simulink model "elec_bipolar_npn_optimised"  (R2018b)
settings: Solver=VariableStepAuto  StartTime=0.0  StopTime=0.04  RelTol=1e-3  AbsTol=1e-3  EnableMultiTasking=on
values from neighbouring files (symbols this model uses):
  fsw = n * 2e3    [Hysteresis.m]    (also in OPtimized.m; SVM.m)
  r = 3    [Hysteresis.m]    (also in OPtimized.m; SVM.m)
libraries: fl_lib x40, nesl_utility x29, elec_lib x12, powerlib_meascontrol x10, simulink x2
settings Model: Creator=Dr. Eskandari  LastModifiedBy=Iftikhw1
settings SolverCC: AutoScaleAbsTol=off
settings DataIOCC: LimitDataPoints=on
settings OptimizationCC: LifeSpan=inf
settings DebuggingCC: AllowSymbolicDim=off  SFUnexpectedBacktrackingDiag=warning  SFNoUnconditionalDefaultTransitionDiag=warning  SFExecutionAtInitializationDiag=none
settings SFSimCC: SimUseLocalCustomCode=off
settings RTWCC: RTWUseLocalCustomCode=off
settings CodeAppCC: StateflowObjectComments=on
settings GRTTargetCC: TargetLangStandard=C89/C90 (ANSI)  GeneratePreprocessorConditionals=Disable all
settings ConfigComp: CovMetricSettings=dw  CovHtmlReporting=on  CovSaveCumulativeToWorkspaceVar=on  CovSaveSingleToWorkspaceVar=on  CovExternalEMLEnable=off  CovSFcnEnable=off
settings SimscapeCC: SimscapeNormalizeSystem=off  SimscapeLogType=all  SimscapeLogDataHistory=10000

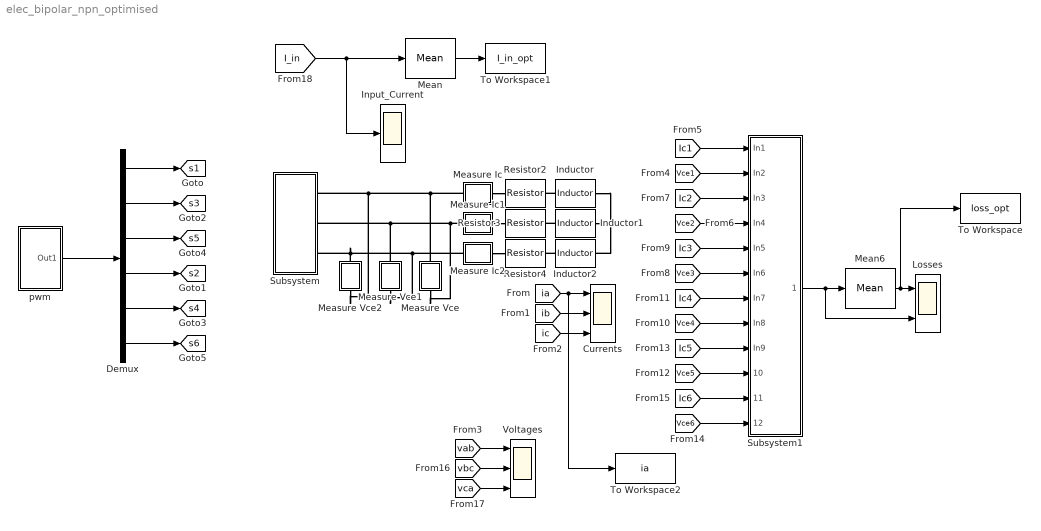
== system elec_bipolar_npn_optimised ==
  Currents : Scope  NumInputPorts=3
  Demux : Demux  Outputs=6
  Inductor : fl_lib/Electrical/Electrical Elements/Inductor  l=1000e-6 H  r=0 Ohm  g=1e-9 1/Ohm  i_specify=off  i_priority=None  i=0 A  i_nominal_specify=off  i_nominal_unit=A  i_nominal_value=1  v_specify=off  v_priority=None  v=0 V  v_nominal_specify=off  v_nominal_unit=V  v_nominal_value=1  i_L_specify=off  i_L_priority=High  i_L=0 A  i_L_nominal_specify=off  i_L_nominal_unit=A  i_L_nominal_value=1
  Inductor1 : fl_lib/Electrical/Electrical Elements/Inductor  l=1000e-6 H  r=0 Ohm  g=1e-9 1/Ohm  i_specify=off  i_priority=None  i=0 A  i_nominal_specify=off  i_nominal_unit=A  i_nominal_value=1  v_specify=off  v_priority=None  v=0 V  v_nominal_specify=off  v_nominal_unit=V  v_nominal_value=1  i_L_specify=off  i_L_priority=High  i_L=0 A  i_L_nominal_specify=off  i_L_nominal_unit=A  i_L_nominal_value=1
  Inductor2 : fl_lib/Electrical/Electrical Elements/Inductor  l=1000e-6 H  r=0 Ohm  g=1e-9 1/Ohm  i_specify=off  i_priority=None  i=0 A  i_nominal_specify=off  i_nominal_unit=A  i_nominal_value=1  v_specify=off  v_priority=None  v=0 V  v_nominal_specify=off  v_nominal_unit=V  v_nominal_value=1  i_L_specify=off  i_L_priority=High  i_L=0 A  i_L_nominal_specify=off  i_L_nominal_unit=A  i_L_nominal_value=1
  Input_Current : Scope
  Losses : Scope  NumInputPorts=2
  Mean : powerlib_meascontrol/Measurements/Mean  Freq=fsw  Vinit=0  Ts=0
  Mean6 : powerlib_meascontrol/Measurements/Mean  Freq=150  Vinit=0  Ts=0
      settings: SourceProductName=Simscape Electrical
  Measure Ic : Subsystem
  Measure Ic1 : Subsystem
  Measure Ic2 : Subsystem
  Measure Vce : Subsystem
  Measure Vce1 : Subsystem
  Measure Vce2 : Subsystem
  Resistor2 : fl_lib/Electrical/Electrical Elements/Resistor  R=r Ohm  i_specify=off  i_priority=None  i=0 A  i_nominal_specify=off  i_nominal_unit=A  i_nominal_value=1  v_specify=off  v_priority=None  v=0 V  v_nominal_specify=off  v_nominal_unit=V  v_nominal_value=1
  Resistor3 : fl_lib/Electrical/Electrical Elements/Resistor  R=r Ohm  i_specify=off  i_priority=None  i=0 A  i_nominal_specify=off  i_nominal_unit=A  i_nominal_value=1  v_specify=off  v_priority=None  v=0 V  v_nominal_specify=off  v_nominal_unit=V  v_nominal_value=1
  Resistor4 : fl_lib/Electrical/Electrical Elements/Resistor  R=r Ohm  i_specify=off  i_priority=None  i=0 A  i_nominal_specify=off  i_nominal_unit=A  i_nominal_value=1  v_specify=off  v_priority=None  v=0 V  v_nominal_specify=off  v_nominal_unit=V  v_nominal_value=1
  Subsystem : Subsystem
  Subsystem1 : Subsystem
  To Workspace : ToWorkspace  VariableName=loss_opt  SampleTime=-1
      settings: MaxDataPoints=1
  To Workspace1 : ToWorkspace  VariableName=I_in_opt  SampleTime=-1
      settings: MaxDataPoints=1
  To Workspace2 : ToWorkspace  VariableName=ia  SampleTime=-1
      settings: MaxDataPoints=1
  Voltages : Scope  NumInputPorts=3
  pwm : Subsystem
  tag scope: s1=global, s2=global, s3=global, s4=global, s5=global, s6=global
  wires:
  Demux/1 -> [s1]
  [ia] -> To Workspace2/1, Currents/1
  [ib] -> Currents/2
  [ic] -> Currents/3
  Mean6/1 -> To Workspace/1, Losses/1
  [Ic1] -> Subsystem1/1(In1)
  [Vce1] -> Subsystem1/2(In2)
  [Ic2] -> Subsystem1/3(In3)
  [Vce2] -> Subsystem1/4(In4)
  [Ic3] -> Subsystem1/5(In5)
  [Vce3] -> Subsystem1/6(In6)
  [Ic4] -> Subsystem1/7(In7)
  [Vce4] -> Subsystem1/8(In8)
  [Ic5] -> Subsystem1/9(In9)
  [Vce5] -> Subsystem1/10(In10)
  [Ic6] -> Subsystem1/11(In11)
  [Vce6] -> Subsystem1/12(In12)
  Subsystem1/1(Out1) -> Losses/2, Mean6/1
  pwm/1(Out1) -> Demux/1
  Demux/4 -> [s2]
  Demux/2 -> [s3]
  Demux/5 -> [s4]
  Demux/3 -> [s5]
  Demux/6 -> [s6]
  [vca] -> Voltages/3
  [vbc] -> Voltages/2
  [vab] -> Voltages/1
  [I_in] -> Input_Current/1, Mean/1
  Mean/1 -> To Workspace1/1
  connections:
  Measure Ic/RConn1 -- Measure Vce/LConn1 -- Measure Vce2/RConn1 -- Subsystem/RConn1
  Measure Ic/LConn1 -- Resistor2/LConn1
  Measure Ic1/RConn1 -- Measure Vce/RConn1 -- Measure Vce1/LConn1 -- Subsystem/RConn2
  Measure Ic1/LConn1 -- Resistor3/LConn1
  Measure Ic2/RConn1 -- Measure Vce1/RConn1 -- Measure Vce2/LConn1 -- Subsystem/RConn3
  Measure Ic2/LConn1 -- Resistor4/LConn1
  Inductor/LConn1 -- Resistor2/RConn1
  Inductor1/LConn1 -- Resistor3/RConn1
  Inductor2/LConn1 -- Resistor4/RConn1
  Inductor/RConn1 -- Inductor1/RConn1 -- Inductor2/RConn1

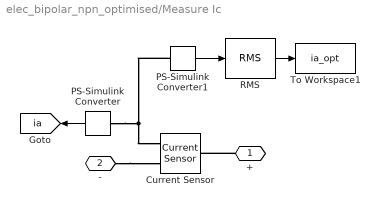
== system elec_bipolar_npn_optimised/Measure Ic ==
  Current Sensor : fl_lib/Electrical/Electrical Sensors/Current Sensor
  PS-Simulink Converter : nesl_utility/PS-Simulink Converter  PhysicalDomain=network_engine_domain  SubClassName=ps_output  LeftPortType=input  RightPortType=output  PseudoPeriodic=off  Frequencies=[]  Unit=1  AffineConversion=off
  PS-Simulink Converter1 : nesl_utility/PS-Simulink Converter  PhysicalDomain=network_engine_domain  SubClassName=ps_output  LeftPortType=input  RightPortType=output  PseudoPeriodic=off  Frequencies=[]  Unit=1  AffineConversion=off
  RMS : powerlib_meascontrol/Measurements/RMS  TrueRMS=off  Freq=50  RMSInit=0  Ts=0
  To Workspace1 : ToWorkspace  VariableName=ia_opt  SampleTime=-1
  + : PMIOPort  Side=Left
  - : PMIOPort  Port=2  Side=Right
  tag scope: ia=global
  wires:
  PS-Simulink Converter/1 -> [ia]
  PS-Simulink Converter1/1 -> RMS/1
  RMS/1 -> To Workspace1/1
  connections:
  +/RConn1 -- Current Sensor/LConn1
  -/RConn1 -- Current Sensor/RConn2
  PS-Simulink Converter/LConn1 -- Current Sensor/RConn1 -- PS-Simulink Converter1/LConn1

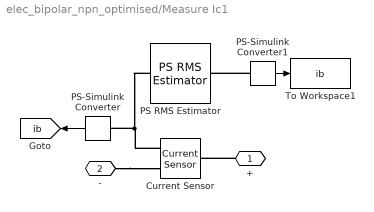
== system elec_bipolar_npn_optimised/Measure Ic1 ==
  Current Sensor : fl_lib/Electrical/Electrical Sensors/Current Sensor
  PS RMS Estimator : fl_lib/Physical Signals/Periodic Operators/PS RMS Estimator  f0=50 Hz
      settings: SourceProductName=Simscape  SourceProductBaseCode=SS
  PS-Simulink Converter : nesl_utility/PS-Simulink Converter  PhysicalDomain=network_engine_domain  SubClassName=ps_output  LeftPortType=input  RightPortType=output  PseudoPeriodic=off  Frequencies=[]  Unit=1  AffineConversion=off
  PS-Simulink Converter1 : nesl_utility/PS-Simulink Converter  PhysicalDomain=network_engine_domain  SubClassName=ps_output  LeftPortType=input  RightPortType=output  PseudoPeriodic=off  Frequencies=[]  Unit=1  AffineConversion=off
  To Workspace1 : ToWorkspace  VariableName=ib  SaveFormat=Timeseries  SampleTime=-1
  + : PMIOPort  Side=Left
  - : PMIOPort  Port=2  Side=Right
  tag scope: ib=global
  wires:
  PS-Simulink Converter/1 -> [ib]
  PS-Simulink Converter1/1 -> To Workspace1/1
  connections:
  Current Sensor/RConn1 -- PS RMS Estimator/LConn1 -- PS-Simulink Converter/LConn1
  -/RConn1 -- Current Sensor/RConn2
  +/RConn1 -- Current Sensor/LConn1
  PS-Simulink Converter1/LConn1 -- PS RMS Estimator/RConn1

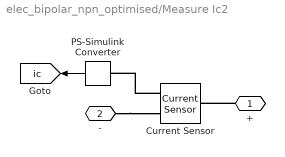
== system elec_bipolar_npn_optimised/Measure Ic2 ==
  Current Sensor : fl_lib/Electrical/Electrical Sensors/Current Sensor
  PS-Simulink Converter : nesl_utility/PS-Simulink Converter  PhysicalDomain=network_engine_domain  SubClassName=ps_output  LeftPortType=input  RightPortType=output  PseudoPeriodic=off  Frequencies=[]  Unit=1  AffineConversion=off
  + : PMIOPort  Side=Left
  - : PMIOPort  Port=2  Side=Right
  tag scope: ic=global
  wires:
  PS-Simulink Converter/1 -> [ic]
  connections:
  +/RConn1 -- Current Sensor/LConn1
  -/RConn1 -- Current Sensor/RConn2
  Current Sensor/RConn1 -- PS-Simulink Converter/LConn1

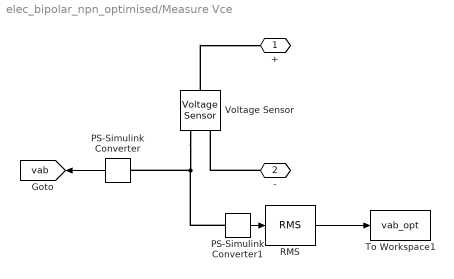
== system elec_bipolar_npn_optimised/Measure Vce ==
  PS-Simulink Converter : nesl_utility/PS-Simulink Converter  PhysicalDomain=network_engine_domain  SubClassName=ps_output  LeftPortType=input  RightPortType=output  PseudoPeriodic=off  Frequencies=[]  Unit=V  AffineConversion=off
  PS-Simulink Converter1 : nesl_utility/PS-Simulink Converter  PhysicalDomain=network_engine_domain  SubClassName=ps_output  LeftPortType=input  RightPortType=output  PseudoPeriodic=off  Frequencies=[]  Unit=1  AffineConversion=off
  RMS : powerlib_meascontrol/Measurements/RMS  TrueRMS=off  Freq=50  RMSInit=0  Ts=0
  To Workspace1 : ToWorkspace  VariableName=vab_opt  SampleTime=-1
  Voltage Sensor : fl_lib/Electrical/Electrical Sensors/Voltage Sensor
  + : PMIOPort  Side=Left
  - : PMIOPort  Port=2  Side=Right
  tag scope: vab=global
  wires:
  PS-Simulink Converter/1 -> [vab]
  PS-Simulink Converter1/1 -> RMS/1
  RMS/1 -> To Workspace1/1
  connections:
  Voltage Sensor/LConn1 -- +/RConn1
  -/RConn1 -- Voltage Sensor/RConn2
  Voltage Sensor/RConn1 -- PS-Simulink Converter1/LConn1 -- PS-Simulink Converter/LConn1

== system elec_bipolar_npn_optimised/Measure Vce1 ==
  PS-Simulink Converter : nesl_utility/PS-Simulink Converter  PhysicalDomain=network_engine_domain  SubClassName=ps_output  LeftPortType=input  RightPortType=output  PseudoPeriodic=off  Frequencies=[]  Unit=V  AffineConversion=off
  Voltage Sensor : fl_lib/Electrical/Electrical Sensors/Voltage Sensor
  + : PMIOPort  Side=Left
  - : PMIOPort  Port=2  Side=Right
  tag scope: vbc=global
  wires:
  PS-Simulink Converter/1 -> [vbc]
  connections:
  Voltage Sensor/RConn1 -- PS-Simulink Converter/LConn1
  -/RConn1 -- Voltage Sensor/RConn2
  Voltage Sensor/LConn1 -- +/RConn1

== system elec_bipolar_npn_optimised/Measure Vce2 ==
  PS-Simulink Converter : nesl_utility/PS-Simulink Converter  PhysicalDomain=network_engine_domain  SubClassName=ps_output  LeftPortType=input  RightPortType=output  PseudoPeriodic=off  Frequencies=[]  Unit=V  AffineConversion=off
  Voltage Sensor : fl_lib/Electrical/Electrical Sensors/Voltage Sensor
  + : PMIOPort  Side=Left
  - : PMIOPort  Port=2  Side=Right
  tag scope: vca=global
  wires:
  PS-Simulink Converter/1 -> [vca]
  connections:
  Voltage Sensor/LConn1 -- +/RConn1
  -/RConn1 -- Voltage Sensor/RConn2
  Voltage Sensor/RConn1 -- PS-Simulink Converter/LConn1

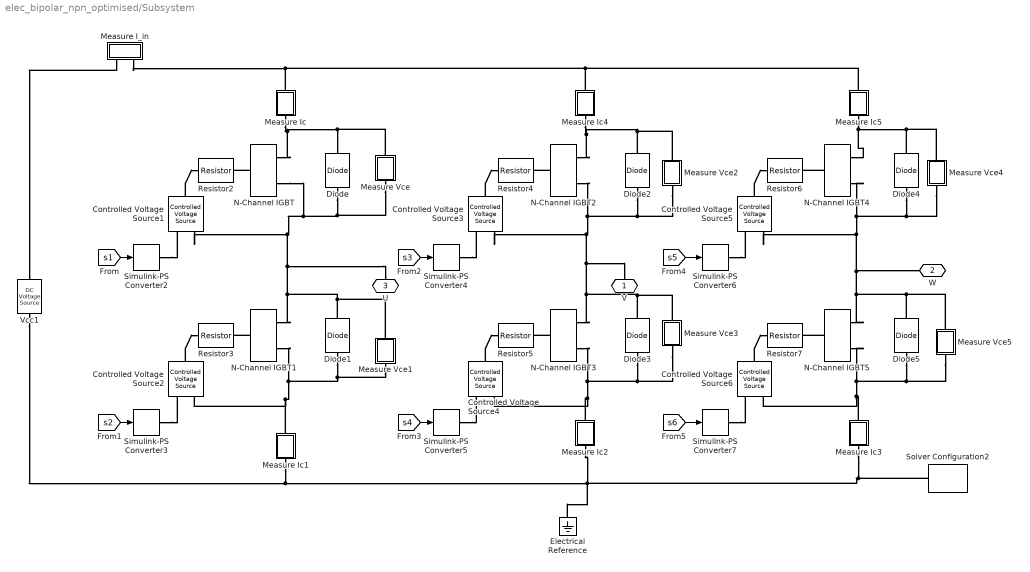
== system elec_bipolar_npn_optimised/Subsystem ==
  Controlled Voltage Source{1..6} (6 alike) : fl_lib/Electrical/Electrical Sources/Controlled Voltage Source
  Diode{,1..5} (6 alike) : elec_lib/Semiconductor Devices/Diode  ModelType=1  Vf=2.15 V  Ron=0.0063 Ohm  Goff=1e-8 S  Rz=0.3 Ohm  Vz=50 V  C_PWL=5 pF  prmExp=1  I12=[ 0.0137 0.545 ] A  V12=[ 0.6 0.7 ] V  I1=0.0137 A  V1=0.6 V  IS=1e-12 A  ec=1  RS=0.01 Ohm  Tmeas=25 degC  BV=Inf V  C_param=1  CJ0=5 pF  VJ=1 V  Mgrad=0.5  Vvec=[ 0.1 10 100 ] V  Cvec=[ 3.5 1 0.4 ] pF  FC=0.5  Q_param=1  Irrm=-7.15 A  iF=4 A  didt=-750 A/us  trr=115 ns  TT=50 ns  tau=100 ns  T_param=1  IS_T2=1.25e-7 A  I1_T2=0.245 A  V1_T2=0.5 V  Tmeas2=125 degC  EG_param=1  EG=1.11 eV  XTI_param=1  XTI=3  dBVdT=0 V/K  Tdevice=25 degC  i_capacitor_specify=off  i_capacitor_priority=High  i_capacitor=0 A  i_capacitor_nominal_specify=off  i_capacitor_nominal_unit=A  i_capacitor_nominal_value=1  v_capacitor_specify=off  v_capacitor_priority=None  v_capacitor=0 V  v_capacitor_nominal_specify=off  v_capacitor_nominal_unit=V  v_capacitor_nominal_value=1  Rth=[ 0 10 ] K/W  thermal_mass_parameterization=1  thermal_mass=[ 0 1 ] J/K  thermal_time_constant=[ 0 10 ] s  thermal_mass_initial_temperatures=[ 25 25 ] degC
      settings: SourceProductName=Simscape Electronics  SourceProductBaseCode=SN
  Electrical Reference : fl_lib/Electrical/Electrical Elements/Electrical Reference
  Measure Ic : Subsystem
  Measure Ic1 : Subsystem
  Measure Ic2 : Subsystem
  Measure Ic3 : Subsystem
  Measure Ic4 : Subsystem
  Measure Ic5 : Subsystem
  Measure Vce : Subsystem
  Measure Vce1 : Subsystem
  Measure Vce2 : Subsystem
  Measure Vce3 : Subsystem
  Measure Vce4 : Subsystem
  Measure Vce5 : Subsystem
  Measure I_in : Subsystem
  N-Channel IGBT{,1..5} (6 alike) : elec_lib/Semiconductor Devices/N-Channel IGBT  model_type=1  Ices=2.6 mA  Vces=1200 V  Vth=5.8 V  Vce_sat=2.05 V  Ice_sat=200 A  Vge_sat=15 V  ec=1  Tmeas=150 degC  Vge_vec=[ -2 6 7 8 10 12 15 20 ] V  Vce_vec=[ -1 0 0.5 1 1.5 2 2.5 3 3.5 4 ] V  T_vec=[25, 125] degC  Ic_mat=[ -1.015e-5 1.35e-8 4.7135e-4 5.092e-4 5.105e-4 5.117500000000001e-4 5.1299e-4 5.1423e-4 5.1548e-4 5.1672e-4; -9.986899999999999e-6 1.35e-8 4.7135e-4 5.092e-4 5.105e-4 5.117500000000001e-4 5.1299e-4 5.1423e-4 5.1548e-4 5.1672e-4; -9.955e-6 1.35e-8 0.0065225 3.3324 48.154 93.661 105.52 105.72 105.93 106.14; -9.955e-6 1.35e-8 0.0065235 3.5783 70.264 166.33 252.4 317.67 353.38 357.39; -9.955e-6 1.35e-8 0.006524 3.7206 89.17100000000001 228.09 371.63 511.02 642.6900000000001 764.04; -9.9549e-6 1.35e-8 0.0065242 3.7716 97.79300000000001 256.21 424.27 592.92 759.2 921.52; -9.9549e-6 1.35e-8 0.0065243 3.8067 104.52 278.11 464.6 654.37 844.5700000000001 1.0339e+3; -9.9549e-6 1.35e-8 0.0065244 3.8324 109.92 295.67 496.54 702.28 909.96 1.1183e+3 ] A  Ic_mat_3D=zeros(8, 10, 2) A  C_param=1  C_GE=23.7 nF  C_GC=2.7 nF  C_CE=0 nF  C_ies=12.5 nF  C_res=0.68 nF  C_oes=0.78 nF  C_GE_vec=[ 25 31 26.5 24.9 25 24.9 24.6 24.7 24.8 ] nF  C_GC_vec=[ 55 9 5.5 3.1 2.5 2.1 1.9 1.8 1.7 ] nF  C_CE_vec=[ 5 11 6.5 4.9 3.5 2.7 2.1 1.7 1.4 ] nF  C_ies_vec=[ 80 40 32 28 27.5 27 26.5 26.5 26.5 ] nF  C_res_vec=[ 55 9 5.5 3.1 2.5 2.1 1.9 1.8 1.7 ] nF  C_oes_vec=[ 60 20 12 8 6 4.8 4 3.5 3.1 ] nF  C_Vce_vec=[ 0 1 2 5 10 15 20 25 30 ] V  charge_linearity_param=1  C_OX=20 nF  V_C_OX=-5 V  TF=82 ns  VAF=200 V  RC=0.001 Ohm  RE=0.001 Ohm  RG=0.001 Ohm  BF=50  T_param=1  Ices_T2=100 mA  EG=1.11 eV  Vce_sat_T2=2.05 V  Tmeas2=150 degC  XTI=3  BEX=-1.5  RG_alpha=0 1/K  Tdevice=25 degC  Tdevice_3D=25 degC  Rth=[0.0, 10.0] K/W  thermal_mass_parameterization=1  thermal_mass=[0.0, 1.0] J/K  thermal_time_constant=[0.0, 10.0] s  thermal_mass_initial_temperatures=[298.15, 298.15] K  Ic_vec1=[0.0, 10.0, 50.0, 100.0, 200.0, 400.0, 600.0] A  Vce_vec1=[0.0, 1.1, 1.3, 1.45, 1.75, 2.25, 2.7] V  Rmiller=0.1 Ohm  Goff=1e-5 1/Ohm  t_on=0.07 us  t_rise=0.7 us  t_off=0.2 us  t_fall=0.5 us  v_meas=300 V  Tj_vec1=[298.15, 398.15] K  Vce_mat1=[0.0, 1.1, 1.3, 1.45, 1.75, 2.25, 2.7; 0.0, 1.0, 1.15, 1.35, 1.7, 2.35, 3.0] V  E_turn_on_mat1=[0.0, 0.2, 1.0, 2.0, 4.0, 8.0, 15.0; 0.0, 0.3, 1.3, 2.5, 5.0, 11.0, 18.0] * 1e-3 J  E_turn_off_mat1=[0.0, 0.3, 1.5, 3.0, 6.0, 15.0, 25.0; 0.0, 0.7, 3.3, 6.5, 13.0, 25.0, 35.0] * 1e-3 J
      settings: SourceProductName=Simscape Electronics  SourceProductBaseCode=SN
  Resistor{2..7} (6 alike) : fl_lib/Electrical/Electrical Elements/Resistor  R=3 Ohm  i_specify=off  i_priority=None  i=0 A  i_nominal_specify=off  i_nominal_unit=A  i_nominal_value=1  v_specify=off  v_priority=None  v=0 V  v_nominal_specify=off  v_nominal_unit=V  v_nominal_value=1
  Simulink-PS Converter{2..7} (6 alike) : nesl_utility/Simulink-PS Converter  PhysicalDomain=network_engine_domain  SubClassName=ps_input  LeftPortType=input  RightPortType=output  PseudoPeriodic=off  Frequencies=[]  NoiseDistribution=none  NoiseParameters=[]  Unit=V  AffineConversion=on  FilteringAndDerivatives=zero  SimscapeFilterOrder=1  InputFilterTimeConstant=.001  UdotUserProvided=1
  Solver Configuration2 : nesl_utility/Solver Configuration  PhysicalDomain=network_engine_domain  SubClassName=solver  LeftPortType=input  RightPortType=generic  Tones=[]  Harmonics=[]  SimulateNoise=off  Profile=off  UseLocalSampling=off  EnableSwitchedLinearOptims=on  FrequencyDomain=off  UseCCode=off  RelTol=0.001  AbsTol=1e-06  MinStep=1e-09  ToWorkspace=off  RevertToSquareIcSolve=off  NumHomotopyIterations=100  PhasorMode=off  PhasorModeNumHarmonics=1  DoDC=on  ResidualTolerance=1e-9  UseLocalSolver=on  LocalSolverChoice=NE_TRAPEZOIDAL_ADVANCER  LocalSolverSampleTime=0.00000001  DoFixedCost=off  MaxNonlinIter=3  MaxModeIter=2  LinearAlgebra=Sparse  EquationFormulation=NE_TIME_EF  DelaysMemoryBudget=1024  AutomaticFiltering=on  FilteringTimeConstant=0.001  PartitionStorageMethod=AS_NEEDED  PartitionMemoryBudget=1024
  Vcc1 : fl_lib/Electrical/Electrical Sources/DC Voltage Source  v0=540 V
  V : PMIOPort  Side=Right
  W : PMIOPort  Port=2  Side=Right
  U : PMIOPort  Port=3  Side=Right
  wires:
  [s1] -> Simulink-PS Converter2/1
  [s6] -> Simulink-PS Converter7/1
  [s2] -> Simulink-PS Converter3/1
  [s3] -> Simulink-PS Converter4/1
  [s4] -> Simulink-PS Converter5/1
  [s5] -> Simulink-PS Converter6/1
  connections:
  Simulink-PS Converter2/RConn1 -- Controlled Voltage Source1/RConn1
  N-Channel IGBT/LConn1 -- Resistor2/RConn1
  Measure Vce2/RConn1 -- Diode2/LConn1 -- N-Channel IGBT2/RConn2 -- V/RConn1 -- N-Channel IGBT3/RConn1 -- Diode3/RConn1 -- Measure Vce3/LConn1 -- Controlled Voltage Source3/RConn2
  Simulink-PS Converter5/RConn1 -- Controlled Voltage Source4/RConn1
  N-Channel IGBT3/LConn1 -- Resistor5/RConn1
  Controlled Voltage Source4/LConn1 -- Resistor5/LConn1
  Simulink-PS Converter4/RConn1 -- Controlled Voltage Source3/RConn1
  Controlled Voltage Source3/LConn1 -- Resistor4/LConn1
  N-Channel IGBT2/LConn1 -- Resistor4/RConn1
  Controlled Voltage Source1/LConn1 -- Resistor2/LConn1
  Controlled Voltage Source2/LConn1 -- Resistor3/LConn1
  N-Channel IGBT1/LConn1 -- Resistor3/RConn1
  Simulink-PS Converter3/RConn1 -- Controlled Voltage Source2/RConn1
  N-Channel IGBT4/LConn1 -- Resistor6/RConn1
  Controlled Voltage Source5/LConn1 -- Resistor6/LConn1
  N-Channel IGBT3/RConn2 -- Diode3/LConn1 -- Measure Vce3/RConn1 -- Measure Ic2/LConn1 -- Controlled Voltage Source4/RConn2
  Simulink-PS Converter6/RConn1 -- Controlled Voltage Source5/RConn1
  Controlled Voltage Source6/LConn1 -- Resistor7/LConn1
  N-Channel IGBT5/LConn1 -- Resistor7/RConn1
  Simulink-PS Converter7/RConn1 -- Controlled Voltage Source6/RConn1
  Measure Ic/LConn1 -- Measure I_in/RConn2 -- Measure Ic5/LConn1 -- Measure Ic4/LConn1
  Diode4/LConn1 -- Measure Vce4/RConn1 -- N-Channel IGBT4/RConn2 -- W/RConn1 -- N-Channel IGBT5/RConn1 -- Diode5/RConn1 -- Measure Vce5/LConn1 -- Controlled Voltage Source5/RConn2
  Measure Vce1/LConn1 -- Diode1/RConn1 -- N-Channel IGBT1/RConn1 -- U/RConn1 -- N-Channel IGBT/RConn2 -- Measure Vce/RConn1 -- Diode/LConn1 -- Controlled Voltage Source1/RConn2
  Measure Ic/RConn1 -- N-Channel IGBT/RConn1 -- Measure Vce/LConn1 -- Diode/RConn1
  Diode1/LConn1 -- Measure Vce1/RConn1 -- N-Channel IGBT1/RConn2 -- Measure Ic1/LConn1 -- Controlled Voltage Source2/RConn2
  Vcc1/RConn1 -- Measure Ic1/RConn1 -- Measure Ic3/RConn1 -- Solver Configuration2/RConn1 -- Measure Ic2/RConn1 -- Electrical Reference/LConn1
  Diode5/LConn1 -- Measure Vce5/RConn1 -- N-Channel IGBT5/RConn2 -- Measure Ic3/LConn1 -- Controlled Voltage Source6/RConn2
  Measure Ic4/RConn1 -- N-Channel IGBT2/RConn1 -- Diode2/RConn1 -- Measure Vce2/LConn1
  Measure Ic5/RConn1 -- N-Channel IGBT4/RConn1 -- Diode4/RConn1 -- Measure Vce4/LConn1
  Measure I_in/RConn1 -- Vcc1/LConn1

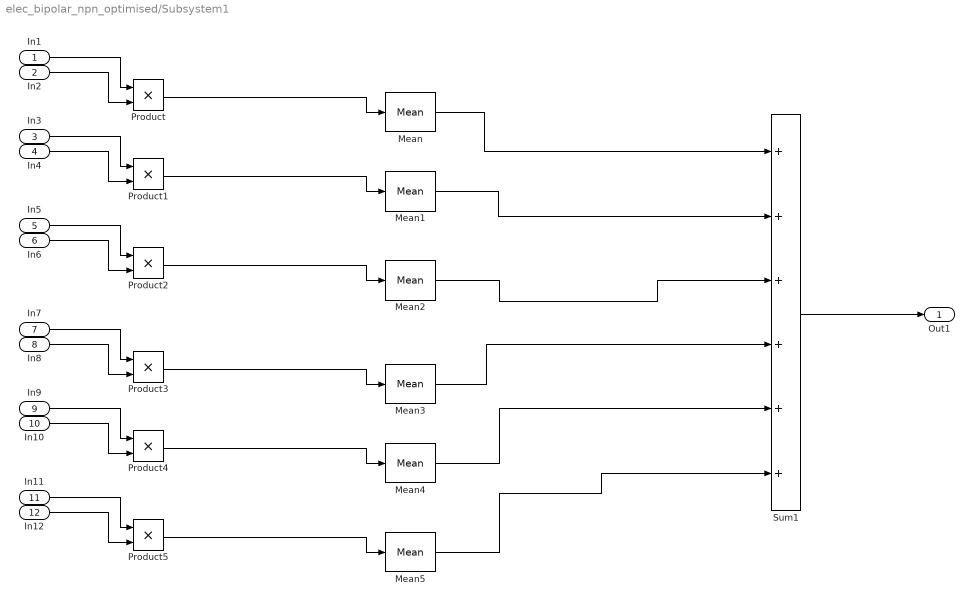
== system elec_bipolar_npn_optimised/Subsystem1 ==
  In1 : Inport
  In2 : Inport  Port=2
  In3 : Inport  Port=3
  In4 : Inport  Port=4
  In5 : Inport  Port=5
  In6 : Inport  Port=6
  In7 : Inport  Port=7
  In8 : Inport  Port=8
  In9 : Inport  Port=9
  In10 : Inport  Port=10
  In11 : Inport  Port=11
  In12 : Inport  Port=12
  Mean{,1..5} (6 alike) : powerlib_meascontrol/Measurements/Mean  Freq=fsw/2  Vinit=0  Ts=0
      settings: SourceProductName=Simscape Electrical
  Product{,1..5} (6 alike) : Product
  Sum1 : Sum  Inputs=++++++
  Out1 : Outport
  wires:
  Product/1 -> Mean/1
  In2/1 -> Product/2
  In1/1 -> Product/1
  Mean/1 -> Sum1/1
  Mean5/1 -> Sum1/6
  Mean1/1 -> Sum1/2
  Product5/1 -> Mean5/1
  In10/1 -> Product4/2
  In4/1 -> Product1/2
  Mean3/1 -> Sum1/4
  In9/1 -> Product4/1
  Mean2/1 -> Sum1/3
  In6/1 -> Product2/2
  In12/1 -> Product5/2
  Product1/1 -> Mean1/1
  In8/1 -> Product3/2
  Product2/1 -> Mean2/1
  Product3/1 -> Mean3/1
  In3/1 -> Product1/1
  In5/1 -> Product2/1
  Mean4/1 -> Sum1/5
  In11/1 -> Product5/1
  In7/1 -> Product3/1
  Sum1/1 -> Out1/1
  Product4/1 -> Mean4/1

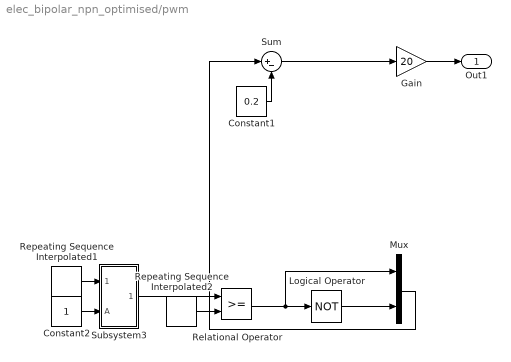
== system elec_bipolar_npn_optimised/pwm ==
  Constant1 : Constant  Value=0.2
  Constant2 : Constant
  Gain : Gain  Gain=20
  Logical Operator : Logic  Operator=NOT  AllPortsSameDT=off  OutDataTypeStr=boolean
  Mux : Mux  Inputs=2
  Relational Operator : RelationalOperator  OutDataTypeStr=boolean  RndMeth=Simplest
  Repeating Sequence Interpolated1 : simulink/Sources/Repeating Sequence Interpolated  OutValues=[0 2*pi].'  TimeValues=[0 0.02].'  LookUpMeth=Interpolation-Use End Values  tsamp=ts  OutMin=[]  OutMax=[]  OutDataTypeStr=double  OutputDataTypeScalingMode=double  OutDataType=fixdt(0,8)  OutScaling=2^-10
  Repeating Sequence Interpolated2 : simulink/Sources/Repeating Sequence Interpolated  OutValues=[0 1].'  TimeValues=[0 1/fsw].'  LookUpMeth=Interpolation-Use End Values  tsamp=ts  OutMin=[]  OutMax=[]  OutDataTypeStr=double  OutputDataTypeScalingMode=double  OutDataType=fixdt(0,8)  OutScaling=2^-10
  Subsystem3 : Subsystem
  Sum : Sum  Inputs=|+-
  Out1 : Outport
  wires:
  Gain/1 -> Out1/1
  Constant1/1 -> Sum/2
  Sum/1 -> Gain/1
  Repeating Sequence Interpolated1/1 -> Subsystem3/1(wt)
  Constant2/1 -> Subsystem3/2(A)
  Subsystem3/1(abc) -> Relational Operator/1
  Repeating Sequence Interpolated2/1 -> Relational Operator/2
  Relational Operator/1 -> Mux/1, Logical Operator/1
  Logical Operator/1 -> Mux/2
  Mux/1 -> Sum/1

== system elec_bipolar_npn_optimised/Subsystem/Measure Ic ==
  Current Sensor : fl_lib/Electrical/Electrical Sensors/Current Sensor
  PS-Simulink Converter : nesl_utility/PS-Simulink Converter  PhysicalDomain=network_engine_domain  SubClassName=ps_output  LeftPortType=input  RightPortType=output  PseudoPeriodic=off  Frequencies=[]  Unit=1  AffineConversion=off
  + : PMIOPort  Side=Left
  - : PMIOPort  Port=2  Side=Right
  tag scope: Ic1=global
  wires:
  PS-Simulink Converter/1 -> [Ic1]
  connections:
  +/RConn1 -- Current Sensor/LConn1
  -/RConn1 -- Current Sensor/RConn2
  Current Sensor/RConn1 -- PS-Simulink Converter/LConn1

== system elec_bipolar_npn_optimised/Subsystem/Measure Ic1 ==
  Current Sensor : fl_lib/Electrical/Electrical Sensors/Current Sensor
  PS-Simulink Converter : nesl_utility/PS-Simulink Converter  PhysicalDomain=network_engine_domain  SubClassName=ps_output  LeftPortType=input  RightPortType=output  PseudoPeriodic=off  Frequencies=[]  Unit=1  AffineConversion=off
  + : PMIOPort  Side=Left
  - : PMIOPort  Port=2  Side=Right
  tag scope: Ic2=global
  wires:
  PS-Simulink Converter/1 -> [Ic2]
  connections:
  +/RConn1 -- Current Sensor/LConn1
  -/RConn1 -- Current Sensor/RConn2
  Current Sensor/RConn1 -- PS-Simulink Converter/LConn1

== system elec_bipolar_npn_optimised/Subsystem/Measure Ic2 ==
  Current Sensor : fl_lib/Electrical/Electrical Sensors/Current Sensor
  PS-Simulink Converter : nesl_utility/PS-Simulink Converter  PhysicalDomain=network_engine_domain  SubClassName=ps_output  LeftPortType=input  RightPortType=output  PseudoPeriodic=off  Frequencies=[]  Unit=1  AffineConversion=off
  + : PMIOPort  Side=Left
  - : PMIOPort  Port=2  Side=Right
  tag scope: Ic4=global
  wires:
  PS-Simulink Converter/1 -> [Ic4]
  connections:
  +/RConn1 -- Current Sensor/LConn1
  -/RConn1 -- Current Sensor/RConn2
  Current Sensor/RConn1 -- PS-Simulink Converter/LConn1

== system elec_bipolar_npn_optimised/Subsystem/Measure Ic3 ==
  Current Sensor : fl_lib/Electrical/Electrical Sensors/Current Sensor
  PS-Simulink Converter : nesl_utility/PS-Simulink Converter  PhysicalDomain=network_engine_domain  SubClassName=ps_output  LeftPortType=input  RightPortType=output  PseudoPeriodic=off  Frequencies=[]  Unit=1  AffineConversion=off
  + : PMIOPort  Side=Left
  - : PMIOPort  Port=2  Side=Right
  tag scope: Ic6=global
  wires:
  PS-Simulink Converter/1 -> [Ic6]
  connections:
  Current Sensor/RConn1 -- PS-Simulink Converter/LConn1
  -/RConn1 -- Current Sensor/RConn2
  +/RConn1 -- Current Sensor/LConn1

== system elec_bipolar_npn_optimised/Subsystem/Measure Ic4 ==
  Current Sensor : fl_lib/Electrical/Electrical Sensors/Current Sensor
  PS-Simulink Converter : nesl_utility/PS-Simulink Converter  PhysicalDomain=network_engine_domain  SubClassName=ps_output  LeftPortType=input  RightPortType=output  PseudoPeriodic=off  Frequencies=[]  Unit=1  AffineConversion=off
  + : PMIOPort  Side=Left
  - : PMIOPort  Port=2  Side=Right
  tag scope: Ic3=global
  wires:
  PS-Simulink Converter/1 -> [Ic3]
  connections:
  +/RConn1 -- Current Sensor/LConn1
  -/RConn1 -- Current Sensor/RConn2
  Current Sensor/RConn1 -- PS-Simulink Converter/LConn1

== system elec_bipolar_npn_optimised/Subsystem/Measure Ic5 ==
  Current Sensor : fl_lib/Electrical/Electrical Sensors/Current Sensor
  PS-Simulink Converter : nesl_utility/PS-Simulink Converter  PhysicalDomain=network_engine_domain  SubClassName=ps_output  LeftPortType=input  RightPortType=output  PseudoPeriodic=off  Frequencies=[]  Unit=1  AffineConversion=off
  + : PMIOPort  Side=Left
  - : PMIOPort  Port=2  Side=Right
  tag scope: Ic5=global
  wires:
  PS-Simulink Converter/1 -> [Ic5]
  connections:
  Current Sensor/RConn1 -- PS-Simulink Converter/LConn1
  -/RConn1 -- Current Sensor/RConn2
  +/RConn1 -- Current Sensor/LConn1

== system elec_bipolar_npn_optimised/Subsystem/Measure Vce ==
  PS-Simulink Converter : nesl_utility/PS-Simulink Converter  PhysicalDomain=network_engine_domain  SubClassName=ps_output  LeftPortType=input  RightPortType=output  PseudoPeriodic=off  Frequencies=[]  Unit=V  AffineConversion=off
  Voltage Sensor : fl_lib/Electrical/Electrical Sensors/Voltage Sensor
  + : PMIOPort  Side=Left
  - : PMIOPort  Port=2  Side=Right
  tag scope: Vce1=global
  wires:
  PS-Simulink Converter/1 -> [Vce1]
  connections:
  Voltage Sensor/LConn1 -- +/RConn1
  -/RConn1 -- Voltage Sensor/RConn2
  Voltage Sensor/RConn1 -- PS-Simulink Converter/LConn1

== system elec_bipolar_npn_optimised/Subsystem/Measure Vce1 ==
  PS-Simulink Converter : nesl_utility/PS-Simulink Converter  PhysicalDomain=network_engine_domain  SubClassName=ps_output  LeftPortType=input  RightPortType=output  PseudoPeriodic=off  Frequencies=[]  Unit=V  AffineConversion=off
  Voltage Sensor : fl_lib/Electrical/Electrical Sensors/Voltage Sensor
  + : PMIOPort  Side=Left
  - : PMIOPort  Port=2  Side=Right
  tag scope: Vce2=global
  wires:
  PS-Simulink Converter/1 -> [Vce2]
  connections:
  Voltage Sensor/RConn1 -- PS-Simulink Converter/LConn1
  -/RConn1 -- Voltage Sensor/RConn2
  Voltage Sensor/LConn1 -- +/RConn1

== system elec_bipolar_npn_optimised/Subsystem/Measure Vce2 ==
  PS-Simulink Converter : nesl_utility/PS-Simulink Converter  PhysicalDomain=network_engine_domain  SubClassName=ps_output  LeftPortType=input  RightPortType=output  PseudoPeriodic=off  Frequencies=[]  Unit=V  AffineConversion=off
  Voltage Sensor : fl_lib/Electrical/Electrical Sensors/Voltage Sensor
  + : PMIOPort  Side=Left
  - : PMIOPort  Port=2  Side=Right
  tag scope: Vce3=global
  wires:
  PS-Simulink Converter/1 -> [Vce3]
  connections:
  Voltage Sensor/LConn1 -- +/RConn1
  -/RConn1 -- Voltage Sensor/RConn2
  Voltage Sensor/RConn1 -- PS-Simulink Converter/LConn1

== system elec_bipolar_npn_optimised/Subsystem/Measure Vce3 ==
  PS-Simulink Converter : nesl_utility/PS-Simulink Converter  PhysicalDomain=network_engine_domain  SubClassName=ps_output  LeftPortType=input  RightPortType=output  PseudoPeriodic=off  Frequencies=[]  Unit=V  AffineConversion=off
  Voltage Sensor : fl_lib/Electrical/Electrical Sensors/Voltage Sensor
  + : PMIOPort  Side=Left
  - : PMIOPort  Port=2  Side=Right
  tag scope: Vce4=global
  wires:
  PS-Simulink Converter/1 -> [Vce4]
  connections:
  Voltage Sensor/RConn1 -- PS-Simulink Converter/LConn1
  -/RConn1 -- Voltage Sensor/RConn2
  Voltage Sensor/LConn1 -- +/RConn1

== system elec_bipolar_npn_optimised/Subsystem/Measure Vce4 ==
  PS-Simulink Converter : nesl_utility/PS-Simulink Converter  PhysicalDomain=network_engine_domain  SubClassName=ps_output  LeftPortType=input  RightPortType=output  PseudoPeriodic=off  Frequencies=[]  Unit=V  AffineConversion=off
  Voltage Sensor : fl_lib/Electrical/Electrical Sensors/Voltage Sensor
  + : PMIOPort  Side=Left
  - : PMIOPort  Port=2  Side=Right
  tag scope: Vce5=global
  wires:
  PS-Simulink Converter/1 -> [Vce5]
  connections:
  Voltage Sensor/RConn1 -- PS-Simulink Converter/LConn1
  -/RConn1 -- Voltage Sensor/RConn2
  Voltage Sensor/LConn1 -- +/RConn1

== system elec_bipolar_npn_optimised/Subsystem/Measure Vce5 ==
  PS-Simulink Converter : nesl_utility/PS-Simulink Converter  PhysicalDomain=network_engine_domain  SubClassName=ps_output  LeftPortType=input  RightPortType=output  PseudoPeriodic=off  Frequencies=[]  Unit=V  AffineConversion=off
  Voltage Sensor : fl_lib/Electrical/Electrical Sensors/Voltage Sensor
  + : PMIOPort  Side=Left
  - : PMIOPort  Port=2  Side=Right
  tag scope: Vce6=global
  wires:
  PS-Simulink Converter/1 -> [Vce6]
  connections:
  Voltage Sensor/LConn1 -- +/RConn1
  -/RConn1 -- Voltage Sensor/RConn2
  Voltage Sensor/RConn1 -- PS-Simulink Converter/LConn1

== system elec_bipolar_npn_optimised/Subsystem/Measure I_in ==
  Current Sensor : fl_lib/Electrical/Electrical Sensors/Current Sensor
  PS-Simulink Converter : nesl_utility/PS-Simulink Converter  PhysicalDomain=network_engine_domain  SubClassName=ps_output  LeftPortType=input  RightPortType=output  PseudoPeriodic=off  Frequencies=[]  Unit=1  AffineConversion=off
  + : PMIOPort  Tag=PMCPort  Side=Right
  - : PMIOPort  Tag=PMCPort  Port=2  Side=Right
  tag scope: I_in=global
  wires:
  PS-Simulink Converter/1 -> [I_in]
  connections:
  Current Sensor/RConn2 -- -/RConn1
  PS-Simulink Converter/LConn1 -- Current Sensor/RConn1
  Current Sensor/LConn1 -- +/RConn1

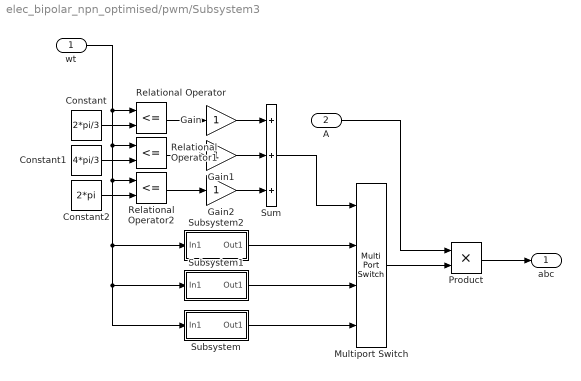
== system elec_bipolar_npn_optimised/pwm/Subsystem3 ==
  wt : Inport
  A : Inport  Port=2
  Constant : Constant  Value=2*pi/3
  Constant1 : Constant  Value=4*pi/3
  Constant2 : Constant  Value=2*pi
  Gain : Gain  OutDataTypeStr=double
  Gain1 : Gain  OutDataTypeStr=double
  Gain2 : Gain  OutDataTypeStr=double
  Multiport Switch : MultiPortSwitch
  Product : Product
  Relational Operator : RelationalOperator  Operator=<=  OutDataTypeStr=boolean  RndMeth=Nearest
  Relational Operator1 : RelationalOperator  Operator=<=  OutDataTypeStr=boolean  RndMeth=Nearest
  Relational Operator2 : RelationalOperator  Operator=<=  OutDataTypeStr=boolean  RndMeth=Nearest
  Subsystem : Subsystem
  Subsystem1 : Subsystem
  Subsystem2 : Subsystem
  Sum : Sum  Inputs=+++
  abc : Outport
  wires:
  Sum/1 -> Multiport Switch/1
  Subsystem2/1(Out1) -> Multiport Switch/2
  Multiport Switch/1 -> Product/2
  Gain/1 -> Sum/1
  wt/1 -> Subsystem2/1(In1), Subsystem/1(In1), Subsystem1/1(In1), Relational Operator2/1, Relational Operator1/1, Relational Operator/1
  Constant/1 -> Relational Operator/2
  Gain2/1 -> Sum/3
  Constant2/1 -> Relational Operator2/2
  Product/1 -> abc/1
  Subsystem1/1(Out1) -> Multiport Switch/3
  Relational Operator/1 -> Gain/1
  Relational Operator1/1 -> Gain1/1
  Relational Operator2/1 -> Gain2/1
  Gain1/1 -> Sum/2
  Subsystem/1(Out1) -> Multiport Switch/4
  Constant1/1 -> Relational Operator1/2
  A/1 -> Product/1

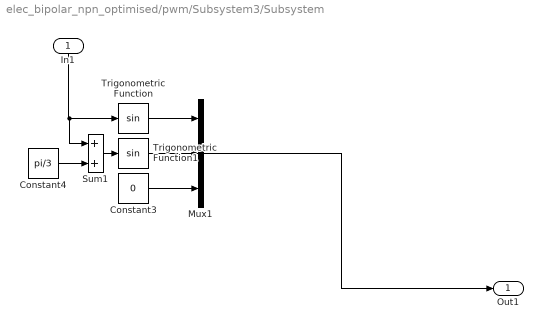
== system elec_bipolar_npn_optimised/pwm/Subsystem3/Subsystem ==
  In1 : Inport
  Constant3 : Constant  Value=0
  Constant4 : Constant  Value=pi/3
  Mux1 : Mux  Inputs=3
  Sum1 : Sum
  Trigonometric Function : Trigonometry
  Trigonometric Function1 : Trigonometry
  Out1 : Outport
  wires:
  Mux1/1 -> Out1/1
  Trigonometric Function/1 -> Mux1/1
  In1/1 -> Sum1/1, Trigonometric Function/1
  Sum1/1 -> Trigonometric Function1/1
  Constant4/1 -> Sum1/2
  Trigonometric Function1/1 -> Mux1/2
  Constant3/1 -> Mux1/3

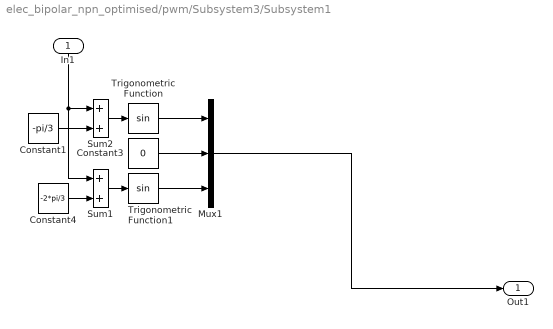
== system elec_bipolar_npn_optimised/pwm/Subsystem3/Subsystem1 ==
  In1 : Inport
  Constant1 : Constant  Value=-pi/3
  Constant3 : Constant  Value=0
  Constant4 : Constant  Value=-2*pi/3
  Mux1 : Mux  Inputs=3
  Sum1 : Sum
  Sum2 : Sum
  Trigonometric Function : Trigonometry
  Trigonometric Function1 : Trigonometry
  Out1 : Outport
  wires:
  Constant4/1 -> Sum1/2
  Sum1/1 -> Trigonometric Function1/1
  In1/1 -> Sum2/1, Sum1/1
  Trigonometric Function/1 -> Mux1/1
  Mux1/1 -> Out1/1
  Constant3/1 -> Mux1/2
  Trigonometric Function1/1 -> Mux1/3
  Sum2/1 -> Trigonometric Function/1
  Constant1/1 -> Sum2/2

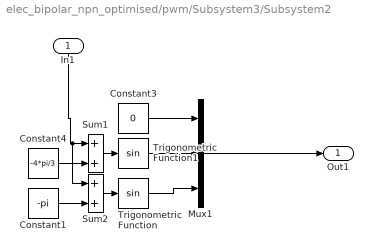
== system elec_bipolar_npn_optimised/pwm/Subsystem3/Subsystem2 ==
  In1 : Inport
  Constant1 : Constant  Value=-pi
  Constant3 : Constant  Value=0
  Constant4 : Constant  Value=-4*pi/3
  Mux1 : Mux  Inputs=3
  Sum1 : Sum
  Sum2 : Sum
  Trigonometric Function : Trigonometry
  Trigonometric Function1 : Trigonometry
  Out1 : Outport
  wires:
  Mux1/1 -> Out1/1
  In1/1 -> Sum2/1, Sum1/1
  Sum1/1 -> Trigonometric Function1/1
  Constant4/1 -> Sum1/2
  Trigonometric Function1/1 -> Mux1/2
  Constant3/1 -> Mux1/1
  Trigonometric Function/1 -> Mux1/3
  Sum2/1 -> Trigonometric Function/1
  Constant1/1 -> Sum2/2
